simulink model "Tractor_Model_Feedforward"  (R2019b)
settings: Solver=FixedStepAuto  StartTime=0.0  StopTime=40  FixedStep=0.01  MaxStep=0.1  RelTol=1e-3
values from neighbouring files (symbols this model uses):
  d = 1    [Tractor_Model.m]    (also in Tractor_Model_Entry.m = 0.4; Tractor_Model_Feedforward_Entry.m = 0.4)
  kD = -5*0.01    (= -0.05)    [Tractor_Model_Entry.m]    (also in Tractor_Model_Feedforward_Entry.m = 0)
  KdPhi = 5*0.01    (= 0.05)    [Tractor_Model_Entry.m]    (also in Tractor_Model_Feedforward_Entry.m = 0.002)
  kPhi = 0.6    [Tractor_Model_Entry.m]    (also in Tractor_Model_Feedforward_Entry.m)
  kX = -0.12    [Tractor_Model_Entry.m]    (also in Tractor_Model_Feedforward_Entry.m = -0.13)
  l = 3    [Tractor_Model.m]    (also in Tractor_Model_Entry.m = 1.72; Tractor_Model_Feedforward_Entry.m = 1.72)
  setPoint = 0    [Tractor_Model_Entry.m]    (also in Tractor_Model_Feedforward_Entry.m)
  stepperAccel = 1.5    [Tractor_Model_Entry.m]    (also in Tractor_Model_Feedforward_Entry.m)
  V2 = 5    [Tractor_Model.m]    (also in Tractor_Model_Entry.m; Tractor_Model_Feedforward_Entry.m = 2.3)
libraries: simulink x1
settings Model: Creator=cessn  LastModifiedBy=cessn

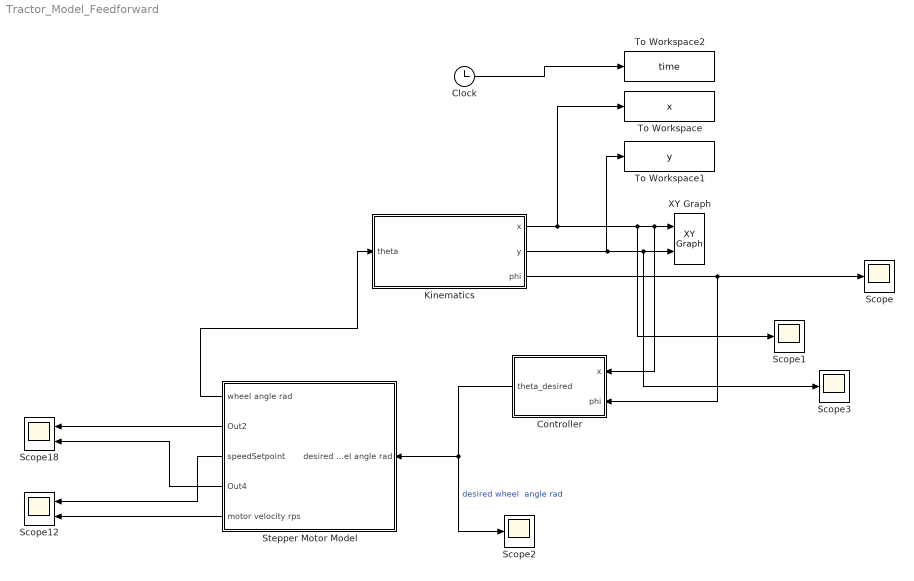
== system Tractor_Model_Feedforward ==
  Clock : Clock
  Controller : Subsystem
  Kinematics : Subsystem
  Scope{,1..3} (4 alike) : Scope
  Scope12 : Scope  NumInputPorts=2
  Scope18 : Scope  NumInputPorts=2
  Stepper Motor Model : Subsystem
  To Workspace : ToWorkspace  VariableName=x  SampleTime=-1
  To Workspace1 : ToWorkspace  VariableName=y  SaveFormat=Timeseries  SampleTime=-1
  To Workspace2 : ToWorkspace  VariableName=time  SampleTime=-1
  XY Graph : simulink/Sinks/XY Graph  xmin=-10  xmax=10  ymin=0  ymax=100  st=-1
  wires:
  Kinematics/1(x) -> Scope1/1, Controller/1(x), XY Graph/1, To Workspace/1
  Kinematics/2(y) -> To Workspace1/1, Scope3/1, XY Graph/2
  Kinematics/3(phi) -> Controller/2(phi), Scope/1
  Controller/1(theta_desired) -> Scope2/1, Stepper Motor Model/1(desired wheel angle rad)  "desired wheel  angle rad"
  Stepper Motor Model/2(Out2) -> Scope18/1
  Stepper Motor Model/3(speedSetpoint) -> Scope12/1
  Stepper Motor Model/4(Out4) -> Scope18/2
  Stepper Motor Model/5(motor velocity rps) -> Scope12/2
  Stepper Motor Model/1(wheel angle rad) -> Kinematics/1(theta)
  Clock/1 -> To Workspace2/1

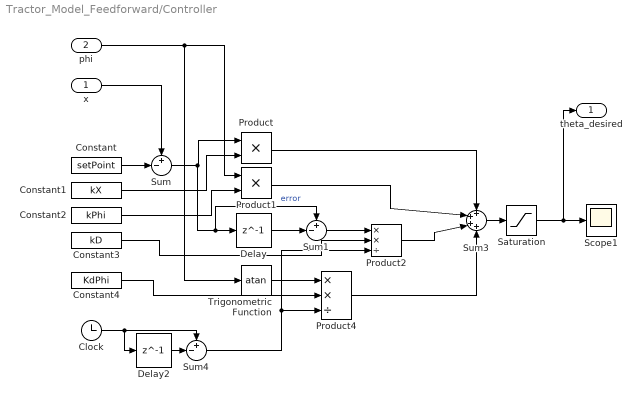
== system Tractor_Model_Feedforward/Controller ==
  x : Inport
  phi : Inport  Port=2
  Clock : Clock
  Constant : Constant  Value=setPoint
  Constant1 : Constant  Value=kX
  Constant2 : Constant  Value=kPhi
  Constant3 : Constant  Value=kD
  Constant4 : Constant  Value=KdPhi
  Delay : Delay  DelayLength=1  InitialCondition=0
  Delay2 : Delay  DelayLength=1  InitialCondition=0
  Product : Product
  Product1 : Product
  Product2 : Product  Inputs=**/
  Product4 : Product  Inputs=**/
  Saturation : Saturate  UpperLimit=0.3  LowerLimit=-0.3
  Scope1 : Scope
  Sum : Sum  Inputs=+-|
  Sum1 : Sum  Inputs=+-|
  Sum3 : Sum  Inputs=++++
  Sum4 : Sum  Inputs=+-|
  Trigonometric Function : Trigonometry  Operator=atan
  theta_desired : Outport
  wires:
  Sum/1 -> Delay/1, Sum1/1, Product/1  "error"
  Product/1 -> Sum3/1
  Sum3/1 -> Saturation/1
  phi/1 -> Trigonometric Function/1, Product1/1
  Delay/1 -> Sum1/2
  Constant1/1 -> Product/2
  Sum1/1 -> Product2/1
  Constant3/1 -> Product2/2
  Product1/1 -> Sum3/2
  Product2/1 -> Sum3/3
  Saturation/1 -> theta_desired/1, Scope1/1
  Constant2/1 -> Product1/2
  Constant/1 -> Sum/2
  x/1 -> Sum/1
  Trigonometric Function/1 -> Product4/1
  Constant4/1 -> Product4/2
  Product4/1 -> Sum3/4
  Clock/1 -> Delay2/1, Sum4/1
  Delay2/1 -> Sum4/2
  Sum4/1 -> Product2/3, Product4/3

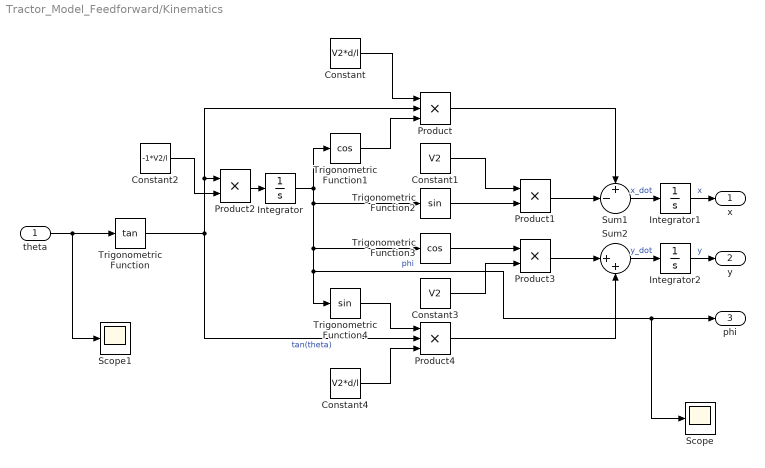
== system Tractor_Model_Feedforward/Kinematics ==
  theta : Inport
  Constant : Constant  Value=V2*d/l
  Constant1 : Constant  Value=V2
  Constant2 : Constant  Value=-1*V2/l
  Constant3 : Constant  Value=V2
  Constant4 : Constant  Value=V2*d/l
  Integrator : Integrator
  Integrator1 : Integrator  InitialCondition=5
  Integrator2 : Integrator
  Product : Product  Inputs=3
  Product1 : Product
  Product2 : Product
  Product3 : Product
  Product4 : Product  Inputs=3
  Scope : Scope
  Scope1 : Scope
  Sum1 : Sum  Inputs=+-|
  Sum2 : Sum  Inputs=|++
  Trigonometric Function : Trigonometry  Operator=tan
  Trigonometric Function1 : Trigonometry  Operator=cos
  Trigonometric Function2 : Trigonometry
  Trigonometric Function3 : Trigonometry  Operator=cos
  Trigonometric Function4 : Trigonometry
  x : Outport
  y : Outport  Port=2
  phi : Outport  Port=3
  wires:
  Trigonometric Function/1 -> Product2/1, Product/2, Product4/2  "tan(theta)"
  Integrator/1 -> Trigonometric Function1/1, Trigonometric Function4/1, Scope/1, phi/1, Trigonometric Function3/1, Trigonometric Function2/1  "phi"
  theta/1 -> Scope1/1, Trigonometric Function/1
  Trigonometric Function2/1 -> Product1/2
  Product/1 -> Sum1/1
  Product1/1 -> Sum1/2
  Product2/1 -> Integrator/1
  Sum2/1 -> Integrator2/1  "y_dot"
  Constant3/1 -> Product3/2
  Sum1/1 -> Integrator1/1  "x_dot"
  Constant/1 -> Product/1
  Product4/1 -> Sum2/2
  Constant1/1 -> Product1/1
  Constant2/1 -> Product2/2
  Trigonometric Function1/1 -> Product/3
  Trigonometric Function4/1 -> Product4/1
  Constant4/1 -> Product4/3
  Product3/1 -> Sum2/1
  Trigonometric Function3/1 -> Product3/1
  Integrator2/1 -> y/1  "y"
  Integrator1/1 -> x/1  "x"

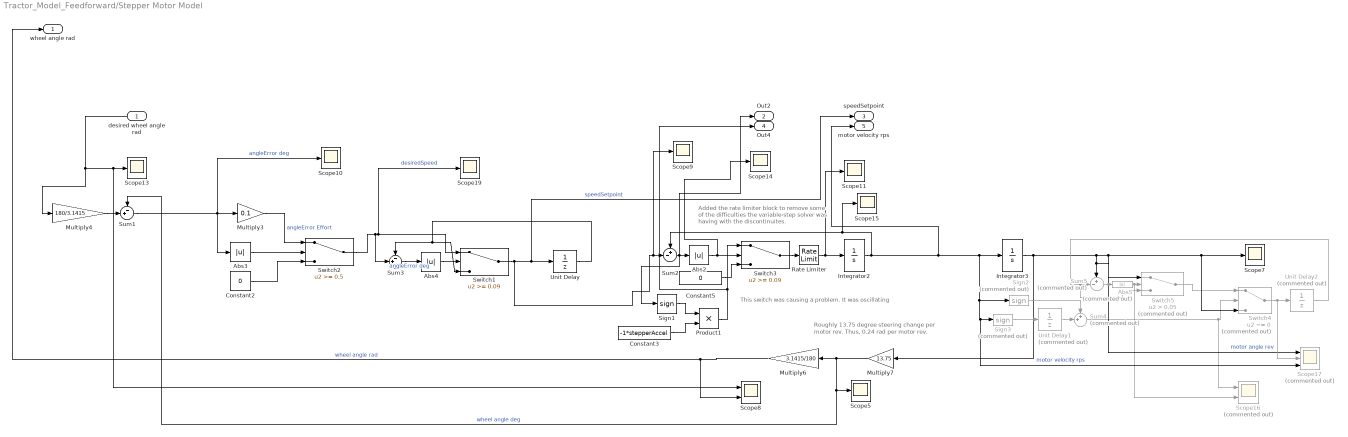
== system Tractor_Model_Feedforward/Stepper Motor Model ==
  note: This switch was causing a problem. It was oscillating
  note: Added the rate limiter block to remove some of the difficulties the variable-step solver was having with the discontinuites.
  note: Roughly 13.75 degree steering change per motor rev. Thus, 0.24 rad per motor rev.
  desired wheel angle rad : Inport
  Abs2 : Abs
  Abs3 : Abs
  Abs4 : Abs
  Abs5 : Abs  Commented=on
  Constant2 : Constant  Value=0
  Constant3 : Constant  Value=-1*stepperAccel
  Constant5 : Constant  Value=0
  Integrator2 : Integrator
  Integrator3 : Integrator
  Multiply3 : Gain  Gain=0.1
  Multiply4 : Gain  Gain=180/3.1415
  Multiply6 : Gain  Gain=3.1415/180
  Multiply7 : Gain  Gain=13.75
  Product1 : Product
  Rate Limiter : RateLimiter  RisingSlewLimit=100  FallingSlewLimit=-100  SampleTimeMode=inherited
  Scope{5,7,9..11,13..15,19} (9 alike) : Scope
  Scope16 : Scope  Commented=on  NumInputPorts=2
  Scope17 : Scope  Commented=on  NumInputPorts=3
  Scope8 : Scope  NumInputPorts=2
  Sign1 : Signum
  Sign2 : Signum  Commented=on
  Sign3 : Signum  Commented=on
  Sum1 : Sum  Inputs=-+|
  Sum2 : Sum  Inputs=+-|
  Sum3 : Sum  Inputs=-+|
  Sum4 : Sum  Commented=on  Inputs=++|
  Sum5 : Sum  Commented=on  Inputs=+-|
  Switch1 : Switch  Threshold=0.09
  Switch2 : Switch  Threshold=0.5
  Switch3 : Switch  Threshold=0.09
  Switch4 : Switch  Commented=on  Criteria=u2 ~= 0
  Switch5 : Switch  Commented=on  Criteria=u2 > Threshold  Threshold=0.05
  Unit Delay : UnitDelay  SampleTime=-1  HasFrameUpgradeWarning=on
  Unit Delay1 : UnitDelay  Commented=on  SampleTime=-1  HasFrameUpgradeWarning=on
  Unit Delay2 : UnitDelay  Commented=on  SampleTime=-1  HasFrameUpgradeWarning=on
  wheel angle rad : Outport
  Out2 : Outport  Port=2
  speedSetpoint : Outport  Port=3
  Out4 : Outport  Port=4
  motor velocity rps : Outport  Port=5
  wires:
  Sum4/1 -> Scope16/1, Switch4/2
  Constant5/1 -> Switch3/3
  Switch5/1 -> Switch4/1
  Abs2/1 -> Scope14/1, Switch3/2
  Abs5/1 -> Scope16/2, Switch5/2
  Integrator3/1 -> Switch5/1, Scope7/1, Switch4/3, Scope17/1, Sum5/1, Multiply7/1  "motor angle rev"
  Integrator2/1 -> Scope15/1, Sum2/1, motor velocity rps/1, Scope17/3, Sign3/1, Sign2/1, Integrator3/1  "motor velocity rps"
  Switch4/1 -> Scope17/2, Unit Delay2/1
  Rate Limiter/1 -> Scope11/1, Integrator2/1
  Sum2/1 -> Out2/1, Sign1/1, Abs2/1
  Multiply7/1 -> Sum1/1, Scope5/1, Multiply6/1  "wheel angle deg"
  Unit Delay2/1 -> Switch5/3, Sum5/2
  Multiply6/1 -> wheel angle rad/1, Scope8/2  "wheel angle rad"
  desired wheel angle rad/1 -> Multiply4/1, Scope8/1, Scope13/1
  Product1/1 -> Out4/1, Switch3/1
  Switch1/1 -> Scope9/1, Sum2/2, speedSetpoint/1, Unit Delay/1  "speedSetpoint"
  Switch2/1 -> Scope19/1, Switch1/1, Sum3/2  "desiredSpeed"
  Multiply4/1 -> Sum1/2
  Multiply3/1 -> Switch2/1  "angleError Effort"
  Sign1/1 -> Product1/1
  Abs3/1 -> Switch2/2
  Constant2/1 -> Switch2/3
  Switch3/1 -> Rate Limiter/1
  Sum3/1 -> Abs4/1  "angleError deg"
  Unit Delay/1 -> Sum3/1, Switch1/3
  Sum5/1 -> Abs5/1
  Constant3/1 -> Product1/2
  Sum1/1 -> Scope10/1, Abs3/1, Multiply3/1  "angleError deg"
  Abs4/1 -> Switch1/2
  Sign3/1 -> Unit Delay1/1
  Unit Delay1/1 -> Sum4/2
  Sign2/1 -> Sum4/1
